simulink model "normal_subject"  (R2021a)
settings: Solver=VariableStepAuto  StartTime=0.0  StopTime=10.0  RelTol=1e-3
libraries: simulink x2
settings Model: Creator=Hansa Niluka  LastModifiedBy=Hansa Niluka

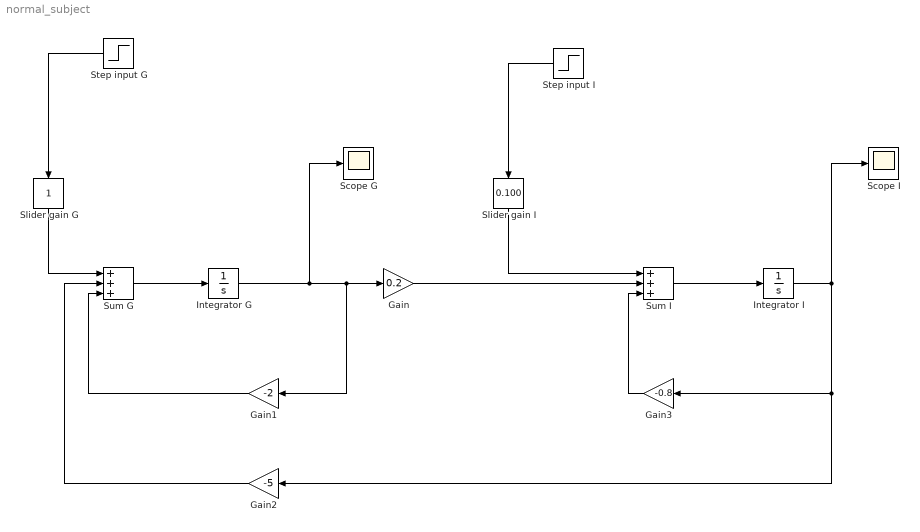
== system normal_subject ==
  Gain : Gain  Gain=0.2
  Gain1 : Gain  Gain=-2
  Gain2 : Gain  Gain=-5
  Gain3 : Gain  Gain=-0.8
  Integrator G : Integrator
  Integrator I : Integrator
  Scope G : Scope
  Scope I : Scope
  Slider gain G : simulink/Math Operations/Slider Gain  gain=1  low=0  high=2
  Slider gain I : simulink/Math Operations/Slider Gain  gain=0.100  low=0  high=2
  Step input G : Step  SampleTime=0
  Step input I : Step  SampleTime=0
  Sum G : Sum  Inputs=+++
  Sum I : Sum  Inputs=+++
  wires:
  Step input I/1 -> Slider gain I/1
  Step input G/1 -> Slider gain G/1
  Gain/1 -> Sum I/2
  Gain1/1 -> Sum G/3
  Sum G/1 -> Integrator G/1
  Sum I/1 -> Integrator I/1
  Gain3/1 -> Sum I/3
  Slider gain G/1 -> Sum G/1
  Integrator G/1 -> Scope G/1, Gain1/1, Gain/1
  Integrator I/1 -> Gain2/1, Gain3/1, Scope I/1
  Gain2/1 -> Sum G/2
  Slider gain I/1 -> Sum I/1
